simulink model "BlocksammlungJan2024"  (R2023b)
settings: Solver=ode45  StartTime=0.0  StopTime=10.0  RelTol=1e-3  EnableMultiTasking=on
undefined symbols (not defined in the file or in its folder): DiscIntNeverNeededParam, Kd, Ki, Kp, ta
libraries: simulink x13, dspxfrm3 x1
(part 2 of 2)

== system BlocksammlungJan2024/PID-Regler2 ==
  w : Inport
  x : Inport  Port=2
  Derivative6 : Derivative
  Integrator5 : Integrator
  Sum : Sum  Inputs=|+-
  Sum9 : Sum  Inputs=+++
  Transfer Fcn : TransferFcn  Denominator=[T 1]
  k_pr1 : Gain  Gain=Ki
  k_pr2 : Gain  Gain=Kp
  k_pr3 : Gain  Gain=Kd
  y : Outport  VectorParamsAs1DForOutWhenUnconnected=off
  wires:
  k_pr3/1 -> Sum9/3  "yd"
  k_pr1/1 -> Sum9/2  "yi"
  Transfer Fcn/1 -> Derivative6/1
  Integrator5/1 -> k_pr1/1
  Sum/1 -> k_pr2/1, Transfer Fcn/1, Integrator5/1
  k_pr2/1 -> Sum9/1  "yp"
  Derivative6/1 -> k_pr3/1
  w/1 -> Sum/1
  Sum9/1 -> y/1
  x/1 -> Sum/2

== system BlocksammlungJan2024/PT1 ==
  u : Inport
  Gain : Gain  Gain=1/T
  Gain1 : Gain  Gain=k
  Integrator : Integrator
  Sum2 : Sum  Inputs=|+-
  v : Outport  VectorParamsAs1DForOutWhenUnconnected=off
  wires:
  u/1 -> Gain1/1
  Sum2/1 -> Gain/1  "T*v'"
  Integrator/1 -> v/1, Sum2/2  "v"
  Gain/1 -> Integrator/1  "v'"
  Gain1/1 -> Sum2/1

== system BlocksammlungJan2024/Schwingkreis ==
  F : Inport
  1/m : Gain  Gain=1/m
  Anfangsgeschwindigkeit : Constant  Value=v0
  Dämpfung : Gain  Gain=D
  Feder : Gain  Gain=C
  Integrator : Integrator
  Integrator1 : Integrator
  Sum : Sum  Inputs=|++
  Sum2 : Sum  Inputs=|+--
  s : Outport  VectorParamsAs1DForOutWhenUnconnected=off
  wires:
  F/1 -> Sum2/1
  Feder/1 -> Sum2/2
  Dämpfung/1 -> Sum2/3
  Sum2/1 -> 1/m/1
  Anfangsgeschwindigkeit/1 -> Sum/2  "[m/s]"
  Sum/1 -> Dämpfung/1, Integrator/1  "v [m/s]"
  Integrator1/1 -> Sum/1
  1/m/1 -> Integrator1/1  "a [m/s2]"
  Integrator/1 -> s/1, Feder/1  "s [m]"

== system BlocksammlungJan2024/Spule ==
  u : Inport
  1dL : Gain  Gain=1/L
  Integrator : Integrator
  i : Outport  VectorParamsAs1DForOutWhenUnconnected=off
  wires:
  u/1 -> Integrator/1  "u"
  1dL/1 -> i/1  "i"
  Integrator/1 -> 1dL/1

== system BlocksammlungJan2024/Spule1 ==
  u : Inport
  1dL : Gain  Gain=1/L
  Integrator : Integrator
  i : Outport  VectorParamsAs1DForOutWhenUnconnected=off
  wires:
  u/1 -> Integrator/1  "u"
  1dL/1 -> i/1  "i"
  Integrator/1 -> 1dL/1

== system BlocksammlungJan2024/SpuleMitDiff ==
  i : Inport
  1dL : Gain  Gain=L
  Derivative : Derivative
  u : Outport  VectorParamsAs1DForOutWhenUnconnected=off
  wires:
  i/1 -> Derivative/1  "i"
  1dL/1 -> u/1  "u"
  Derivative/1 -> 1dL/1  "i'"

== system BlocksammlungJan2024/SpuleMitDiff1 ==
  i : Inport
  1dL : Gain  Gain=L
  Derivative : Derivative
  u : Outport  VectorParamsAs1DForOutWhenUnconnected=off
  wires:
  i/1 -> Derivative/1  "i"
  1dL/1 -> u/1  "u"
  Derivative/1 -> 1dL/1  "i'"

== system BlocksammlungJan2024/Subsystem1 ==
  Trigger : TriggerPort  VariantControl=Variant  PortDimensions=1
  Compare To Constant : simulink/Logic and Bit Operations/Compare To Constant  relop=>=  const=Maximum  OutDataTypeStr=boolean
  Constant : Constant
  Delay : Delay  DelayLength=1  InitialCondition=-1  ExternalReset=Rising
      settings: InputPortMap=u0,r5
  Delay1 : Delay  DelayLength=1
  Sum : Sum  Inputs=|++
  Out1 : Outport  VectorParamsAs1DForOutWhenUnconnected=off
  wires:
  Constant/1 -> Sum/1
  Delay1/1 -> Compare To Constant/1
  Sum/1 -> Out1/1, Delay1/1, Delay/1
  Delay/1 -> Sum/2
  Compare To Constant/1 -> Delay/2

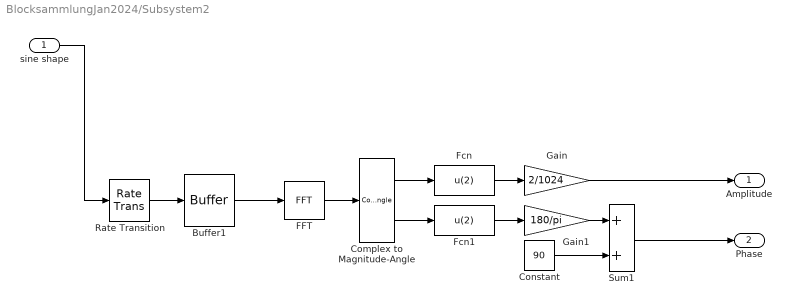
== system BlocksammlungJan2024/Subsystem2 ==
  sine shape : Inport
  Buffer1 : Buffer  N=1024  OutputFrames=off
  Complex to Magnitude-Angle : ComplexToMagnitudeAngle
  Constant : Constant  Value=90
  FFT : dspxfrm3/FFT  FFTImplementation=Auto  CompMethod=Table lookup  TableOpt=NEW  TableOptActive=Speed  BitRevOrder=off  Normalize=off  InheritFFTLength=on  FFTLength=64  WrapInput=on  roundingMode=Floor  overflowMode=off  firstCoeffDataTypeStr=Inherit: Same word length as input  firstCoeffLastDataTypeStr=Inherit: Same word length as input  outputMin=[]  outputMax=[]
  Fcn : Fcn  Expr=u(2)
  Fcn1 : Fcn  Expr=u(2)
  Gain : Gain  Gain=2/1024
  Gain1 : Gain  Gain=180/pi
  Rate Transition : RateTransition  OutPortSampleTime=1/f/1024
  Sum1 : Sum
  Amplitude : Outport  VectorParamsAs1DForOutWhenUnconnected=off
  Phase : Outport  Port=2  VectorParamsAs1DForOutWhenUnconnected=off
  wires:
  sine shape/1 -> Rate Transition/1
  Sum1/1 -> Phase/1
  Constant/1 -> Sum1/2
  Fcn/1 -> Gain/1
  Complex to Magnitude-Angle/1 -> Fcn/1
  Buffer1/1 -> FFT/1
  Gain/1 -> Amplitude/1
  Complex to Magnitude-Angle/2 -> Fcn1/1
  Fcn1/1 -> Gain1/1
  Rate Transition/1 -> Buffer1/1
  Gain1/1 -> Sum1/1
  FFT/1 -> Complex to Magnitude-Angle/1

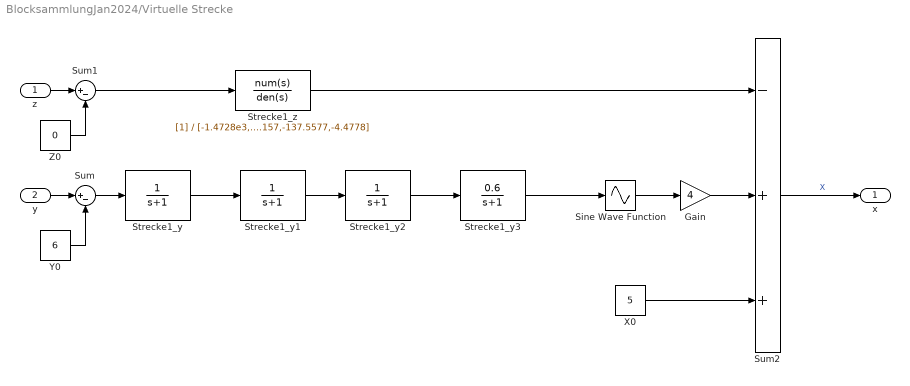
== system BlocksammlungJan2024/Virtuelle Strecke ==
  z : Inport
  y : Inport  Port=2
  Gain : Gain  Gain=4
  Sine Wave Function : Sin  TimeSource=Use external signal  SampleTime=0
  Strecke1_y : TransferFcn  Denominator=[1,1]
  Strecke1_y1 : TransferFcn  Denominator=[1,1]
  Strecke1_y2 : TransferFcn  Denominator=[1,1]
  Strecke1_y3 : TransferFcn  Numerator=[0.6]  Denominator=[1,1]
  Strecke1_z : TransferFcn  Denominator=[-1.4728e3,-534.157,-137.5577,-4.4778]
  Sum : Sum  Inputs=|+-
  Sum1 : Sum  Inputs=|+-
  Sum2 : Sum  Inputs=-++
  X0 : Constant  Value=5
  Y0 : Constant  Value=6
  Z0 : Constant  Value=0
  x : Outport  VectorParamsAs1DForOutWhenUnconnected=off
  wires:
  Sum2/1 -> x/1  "X"
  y/1 -> Sum/1
  z/1 -> Sum1/1
  X0/1 -> Sum2/3
  Strecke1_z/1 -> Sum2/1
  Z0/1 -> Sum1/2
  Sum1/1 -> Strecke1_z/1
  Y0/1 -> Sum/2
  Sum/1 -> Strecke1_y/1
  Strecke1_y/1 -> Strecke1_y1/1
  Strecke1_y1/1 -> Strecke1_y2/1
  Strecke1_y2/1 -> Strecke1_y3/1
  Strecke1_y3/1 -> Sine Wave Function/1
  Sine Wave Function/1 -> Gain/1
  Gain/1 -> Sum2/2

== system BlocksammlungJan2024/Widerstand ==
  i : Inport
  1/m : Gain  Gain=R
  u : Outport  VectorParamsAs1DForOutWhenUnconnected=off
  wires:
  i/1 -> 1/m/1  "i"
  1/m/1 -> u/1  "u"

== system BlocksammlungJan2024/Widerstand1 ==
  i : Inport
  1/m : Gain  Gain=R
  u : Outport  VectorParamsAs1DForOutWhenUnconnected=off
  wires:
  i/1 -> 1/m/1  "i"
  1/m/1 -> u/1  "u"

== system BlocksammlungJan2024/Widerstand2 ==
  i : Inport
  1/m : Gain  Gain=1/R
  u : Outport  VectorParamsAs1DForOutWhenUnconnected=off
  wires:
  i/1 -> 1/m/1  "i"
  1/m/1 -> u/1  "u"

== system BlocksammlungJan2024/Widerstand3 ==
  u : Inport
  1dR : Gain  Gain=1/R
  i : Outport  VectorParamsAs1DForOutWhenUnconnected=off
  wires:
  u/1 -> 1dR/1  "u"
  1dR/1 -> i/1  "i"

== system BlocksammlungJan2024/Industrieregler/DT1 ==
  note: Beim Umschalten von Hand auf Automatik wird de genull. Vorher hatte de einen bliebigen Wert.
      | Somit ergibt sich eine sehr starke Änderung, deren Ableitung dann einen sehr hohen Wert ergibt.
      | Deshalb wird das Umschalten um einen Simulationsschritt verzögert.
      | Somit wird der durch das Umschalten bedingte Peak nicht auf das PT1 Glied gegeben.
  auto : Inport
  kd_mal_de : Inport  Port=2
  Delay1 : Delay  DelayLength=1
  Derivative : Derivative
  Switch3 : Switch  Threshold=0.5  SaturateOnIntegerOverflow=off  InputSameDT=off
  Transfer Fcn : TransferFcn  Denominator=[T 1]
  Y3 : Constant  Value=0
  Out1 : Outport  VectorParamsAs1DForOutWhenUnconnected=off
  wires:
  Delay1/1 -> Switch3/2
  auto/1 -> Delay1/1
  Derivative/1 -> Switch3/1
  kd_mal_de/1 -> Derivative/1
  Switch3/1 -> Transfer Fcn/1
  Y3/1 -> Switch3/3
  Transfer Fcn/1 -> Out1/1  "realer D-Anteil"

== system BlocksammlungJan2024/Industrieregler/Schreibe Y0 zurück ==
  In1 : Inport
  Trigger : TriggerPort  TriggerType=falling  VariantControl=Variant
  MATLAB Function : MATLAB Function  TreatAsAtomicUnit=on
  wires:
  In1/1 -> MATLAB Function/1(u)

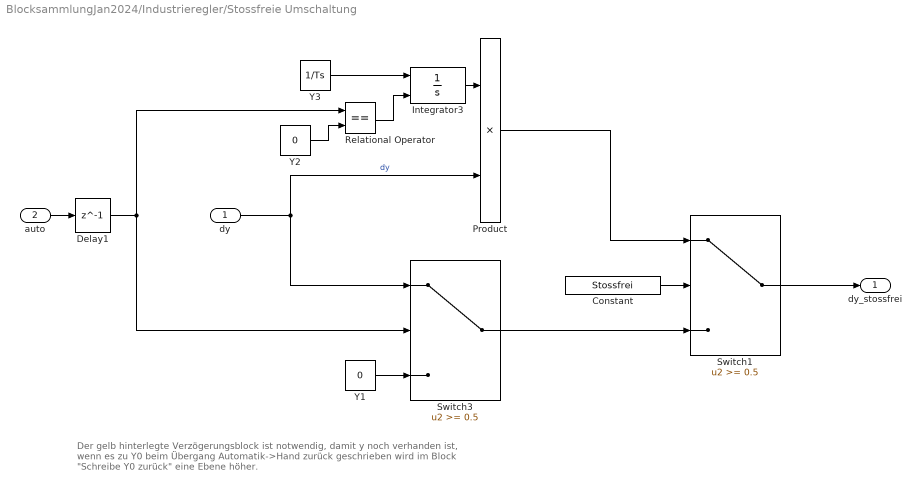
== system BlocksammlungJan2024/Industrieregler/Stossfreie Umschaltung ==
  note: Der gelb hinterlegte Verzögerungsblock ist notwendig, damit y noch verhanden ist, wenn es zu Y0 beim Übergang Automatik->Hand zurück geschrieben wird im Block "Schreibe Y0 zurück" eine Ebene höher.
  dy : Inport
  auto : Inport  Port=2
  Constant : Constant  Value=Stossfrei
  Delay1 : Delay  DelayLength=1
  Integrator3 : Integrator  ExternalReset=level  LimitOutput=on  UpperSaturationLimit=1
      settings: AttributesFormatString=max=%<LimitOutput>
  Product : Product
  Relational Operator : RelationalOperator  Operator===  OutDataTypeStr=boolean  RndMeth=Simplest  InputSameDT=off
  Switch1 : Switch  Threshold=0.5  SaturateOnIntegerOverflow=off  InputSameDT=off
  Switch3 : Switch  Threshold=0.5  SaturateOnIntegerOverflow=off  InputSameDT=off
  Y1 : Constant  Value=0
  Y2 : Constant  Value=0
  Y3 : Constant  Value=1/Ts
  dy_stossfrei : Outport  VectorParamsAs1DForOutWhenUnconnected=off
  wires:
  Integrator3/1 -> Product/1
  Switch1/1 -> dy_stossfrei/1
  Constant/1 -> Switch1/2
  Switch3/1 -> Switch1/3
  Product/1 -> Switch1/1
  Y1/1 -> Switch3/3
  Delay1/1 -> Relational Operator/1, Switch3/2
  dy/1 -> Product/2, Switch3/1  "dy"
  Y2/1 -> Relational Operator/2
  Relational Operator/1 -> Integrator3/2
  auto/1 -> Delay1/1
  Y3/1 -> Integrator3/1

== system BlocksammlungJan2024/Industrieregler/Triggered Subsystem ==
  In1 : Inport
  Trigger : TriggerPort  VariantControl=Variant
  Out1 : Outport  VectorParamsAs1DForOutWhenUnconnected=off
  wires:
  In1/1 -> Out1/1

== system BlocksammlungJan2024/Industrieregler/Triggered Subsystem1 ==
  In1 : Inport
  Trigger : TriggerPort  VariantControl=Variant
  Out1 : Outport  VectorParamsAs1DForOutWhenUnconnected=off
  wires:
  In1/1 -> Out1/1

== system BlocksammlungJan2024/Industrieregler diskret/DT1 ==
  note: Beim Umschalten von Hand auf Automatik wird de genull. Vorher hatte de einen bliebigen Wert.
      | Somit ergibt sich eine sehr starke Änderung, deren Ableitung dann einen sehr hohen Wert ergibt.
      | Deshalb wird das Umschalten um einen Simulationsschritt verzögert.
      | Somit wird der durch das Umschalten bedingte Peak nicht auf das PT1 Glied gegeben.
  auto : Inport
  kd_mal_de : Inport  Port=2
  Delay1 : Delay  DelayLength=1
  Discrete Derivative : simulink/Discrete/Discrete Derivative  gainval=1.0  ICPrevScaledInput=0.0  OutMin=[]  OutMax=[]  OutDataType=fixdt(1, 16)  OutScaling=2^-10  DoSatur=off
  PT1 : DiscreteTransferFcn  Numerator=[1-exp(-ta/T) 0]  Denominator=[1 -exp(-ta/T)]  SampleTime=ta
  Switch3 : Switch  Threshold=0.5  SaturateOnIntegerOverflow=off  InputSameDT=off
  Y3 : Constant  Value=0
  Out1 : Outport  VectorParamsAs1DForOutWhenUnconnected=off
  wires:
  PT1/1 -> Out1/1  "realer D-Anteil"
  Y3/1 -> Switch3/3
  Switch3/1 -> PT1/1
  kd_mal_de/1 -> Discrete Derivative/1
  Discrete Derivative/1 -> Switch3/1
  auto/1 -> Delay1/1
  Delay1/1 -> Switch3/2

== system BlocksammlungJan2024/Industrieregler diskret/Schreibe Y0 zurück ==
  In1 : Inport
  Trigger : TriggerPort  TriggerType=falling  VariantControl=Variant
  MATLAB Function : MATLAB Function  TreatAsAtomicUnit=on
  wires:
  In1/1 -> MATLAB Function/1(u)

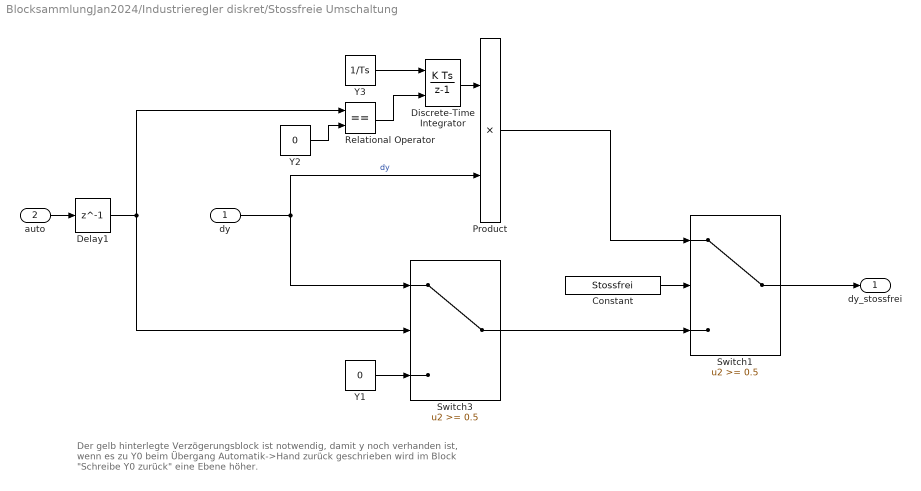
== system BlocksammlungJan2024/Industrieregler diskret/Stossfreie Umschaltung ==
  note: Der gelb hinterlegte Verzögerungsblock ist notwendig, damit y noch verhanden ist, wenn es zu Y0 beim Übergang Automatik->Hand zurück geschrieben wird im Block "Schreibe Y0 zurück" eine Ebene höher.
  dy : Inport
  auto : Inport  Port=2
  Constant : Constant  Value=Stossfrei
  Delay1 : Delay  DelayLength=1
  Discrete-Time Integrator : DiscreteIntegrator  ExternalReset=level  SampleTime=ta  LimitOutput=on  UpperSaturationLimit=1  ICPrevOutput=DiscIntNeverNeededParam  ICPrevScaledInput=DiscIntNeverNeededParam
  Product : Product
  Relational Operator : RelationalOperator  Operator===  OutDataTypeStr=boolean  RndMeth=Simplest  InputSameDT=off
  Switch1 : Switch  Threshold=0.5  SaturateOnIntegerOverflow=off  InputSameDT=off
  Switch3 : Switch  Threshold=0.5  SaturateOnIntegerOverflow=off  InputSameDT=off
  Y1 : Constant  Value=0
  Y2 : Constant  Value=0
  Y3 : Constant  Value=1/Ts
  dy_stossfrei : Outport  VectorParamsAs1DForOutWhenUnconnected=off
  wires:
  Y3/1 -> Discrete-Time Integrator/1
  auto/1 -> Delay1/1
  Relational Operator/1 -> Discrete-Time Integrator/2
  Y2/1 -> Relational Operator/2
  dy/1 -> Switch3/1, Product/2  "dy"
  Delay1/1 -> Switch3/2, Relational Operator/1
  Y1/1 -> Switch3/3
  Product/1 -> Switch1/1
  Switch3/1 -> Switch1/3
  Constant/1 -> Switch1/2
  Switch1/1 -> dy_stossfrei/1
  Discrete-Time Integrator/1 -> Product/1

== system BlocksammlungJan2024/Industrieregler diskret/Triggered Subsystem ==
  In1 : Inport
  Trigger : TriggerPort  VariantControl=Variant
  Out1 : Outport  VectorParamsAs1DForOutWhenUnconnected=off
  wires:
  In1/1 -> Out1/1

== system BlocksammlungJan2024/Industrieregler diskret/Triggered Subsystem1 ==
  In1 : Inport
  Trigger : TriggerPort  VariantControl=Variant
  Out1 : Outport  VectorParamsAs1DForOutWhenUnconnected=off
  wires:
  In1/1 -> Out1/1

== matlab function BlocksammlungJan2024/Industrieregler diskret/Schreibe Y0 zurück/MATLAB Function ==
  data: u input
function  fcn(u)
%#codegen
coder.extrinsic('set_param')
coder.extrinsic('num2str')
coder.extrinsic('bdroot')
coder.extrinsic('get_param')
coder.extrinsic('gcbh')
coder.extrinsic('gcb')
coder.extrinsic('findstr')
coder.extrinsic('length')
%My_ModelWorkSpace = get_param('C1','ModelWorkSpace')
%My_ModelWorkSpace.assignin('U0', u)
%An awefull lot of code just to move two hirachy steps up...
string='This is just a string that is considered to have enough characters for whatever we want to do with the variable test later down the road let us add somme additional characters like abcdefg and hope that this is enough right now This is just a string that is considered to have enough characters for whatever we want to do with the variable test later down the road let us add somme additional characters like abcdefg and hope that this is enough right now This is just a string that is considered to have enough characters for whatever we want to do with the variable test later down the road let us add somme additional characters like abcdefg and hope that this is enough right now This is just a string that is considered to have enough characters for whatever we want to do with the variable test later down the road let us add somme additional characters like abcdefg and hope that this is enough right now This is just a string that is considered to have enough characters for whatever we want to do with the variable test later down the road let us add somme additional characters like abcdefg and hope that this is enough right now This is just a string that is considered to have enough characters for whatever we want to do with the variable test later down the road let us add somme additional characters like abcdefg and hope that this is enough right now This is just a string that is considered to have enough characters for whatever we want to do with the variable test later down the road let us add somme additional characters like abcdefg and hope that this is enough right now This is just a string that is considered to have enough characters for whatever we want to do with the variable test later down the road let us add somme additional characters like abcdefg and hope that this is enough right now'
Length=uint8(1)
Length=uint8(length(gcb))
string(1:Length)=gcb
index=uint8(1)
index=uint8(strfind(gcb,'industrial controller'))
set_param([string(1:index-1),'Y0'],'Value',num2str(u))
end

== matlab function BlocksammlungJan2024/MATLAB Function1 ==
function RT_Pacer
coder.extrinsic('tic') 
coder.extrinsic('toc') 
coder.extrinsic('bdroot')
coder.extrinsic('get_param') 
coder.extrinsic('eval')
coder.extrinsic('disp')
coder.extrinsic('set_param')
tic
time=double(0);
SolverType='Ein Text mit Zeichen';

if ~contains(get_param(bdroot, 'SolverType'),"Fixed-step") 
    fprintf(2,'%s','Real Time Pacer ist nur für fixed step gedacht, Simmulation wurde beendet')
    set_param(bdroot, 'SimulationCommand', 'stop')
end
fundamentalSampleTime=double(1);
fundamentalSampleTime=eval(get_param(bdroot,'FixedStep'));
time=double(toc);
while time<=fundamentalSampleTime
pause(0.0001)
time=double(toc);
end

== matlab function BlocksammlungJan2024/MATLAB Function ==
  data: u input; y output
function y = fcn(u)

y = u;

== matlab function BlocksammlungJan2024/Industrieregler/Schreibe Y0 zurück/MATLAB Function ==
  data: u input
function  fcn(u)
%#codegen
coder.extrinsic('set_param')
coder.extrinsic('num2str')
coder.extrinsic('bdroot')
coder.extrinsic('get_param')
coder.extrinsic('gcbh')
coder.extrinsic('gcb')
coder.extrinsic('findstr')
coder.extrinsic('length')
%My_ModelWorkSpace = get_param('C1','ModelWorkSpace')
%My_ModelWorkSpace.assignin('U0', u)
%An awefull lot of code just to move two hirachy steps up...
string='This is just a string that is considered to have enough characters for whatever we want to do with the variable test later down the road let us add somme additional characters like abcdefg and hope that this is enough right now This is just a string that is considered to have enough characters for whatever we want to do with the variable test later down the road let us add somme additional characters like abcdefg and hope that this is enough right now This is just a string that is considered to have enough characters for whatever we want to do with the variable test later down the road let us add somme additional characters like abcdefg and hope that this is enough right now This is just a string that is considered to have enough characters for whatever we want to do with the variable test later down the road let us add somme additional characters like abcdefg and hope that this is enough right now This is just a string that is considered to have enough characters for whatever we want to do with the variable test later down the road let us add somme additional characters like abcdefg and hope that this is enough right now This is just a string that is considered to have enough characters for whatever we want to do with the variable test later down the road let us add somme additional characters like abcdefg and hope that this is enough right now This is just a string that is considered to have enough characters for whatever we want to do with the variable test later down the road let us add somme additional characters like abcdefg and hope that this is enough right now This is just a string that is considered to have enough characters for whatever we want to do with the variable test later down the road let us add somme additional characters like abcdefg and hope that this is enough right now'
Length=uint8(1)
Length=uint8(length(gcb))
string(1:Length)=gcb
index=uint8(1)
index=uint8(strfind(gcb,'Industrieregler'))
set_param([string(1:index-1),'Y0'],'Value',num2str(u))
end
